simulink model "Copy_of_FaultFeeder"  (R2019a)
settings: Solver=ode1  StartTime=0.0  StopTime=2.5  FixedStep=Ts_Power  RelTol=1e-3
PostLoadFcn:
  | %% Init for wind PnO models - global system parameters
  | OVERRIDE_SSN_MEMORY_LIMIT=1;
  | Ts=50e-6;
  | % Ts=50e-10;
  | Ts_Power=Ts;
  | Ts_Control=2*Ts;
  | freq = 50;
  | Fnom=freq;
  | Vac=400e3;
InitFcn:
  | %% Init for wind PnO models - global system parameters
  | OVERRIDE_SSN_MEMORY_LIMIT=1;
  | Ts=50e-6;
  | % Ts=50e-10;
  | Ts_Power=Ts;
  | Ts_Control=2*Ts;
  | freq = 50;
  | Fnom=freq;
  | Vac=225e3;
values from neighbouring files (symbols this model uses):
  sub_posCap = sub_posCap*2.5    (= 4e-07)    [variable.m]
  sub_posInd = 0.001400563    [variable.m]
  sub_posR = 0.036    [variable.m]
  sub_zeroCap = sub_zeroCap*2.5    (= 1.333325e-07)    [variable.m]
  sub_zeroInd = 0.00420169    [variable.m]
  sub_zeroR = 0.108    [variable.m]
  transfo_L1 = 0.05999374    [variable.m]
  transfo_L2 = 0.05999374    [variable.m]
  transfo_R1 = 0.000866667    [variable.m]
  transfo_R2 = 0.00086667    [variable.m]
undefined symbols (not defined in the file or in its folder): D1, D11, Delta, den, DiscIntNeverNeededParam, dx, find_system, gcbh, num, out_Buses, out_WindFarms, sps_rtmsupport
libraries: powerlib x137, simulink x64, powerlib_meascontrol x64, elements x52, simulink_extras x38, eeSinusoidalMeasurement x35, spsVIMeasurementModel x27, eePowerMeasurement x11
(part 6 of 20)

== system Copy_of_FaultFeeder/SM_WT1/Impedance Element 1/Impedance Relay Scheme ==
  note: Impedance Relay Scheme
  Vabc : Inport
  Iabc : Inport  Port=2
  " 7" : Product  RndMeth=Zero
  "Analog filtering, signal conditioning" : Subsystem
  Combination of Voltages and Currents into 6 pairs (for each type of fault) : Subsystem
  DFT delay : TransportDelay  DelayTime=0.017  BufferSize=30720
  Fault A-B-C Measurement : Subsystem
  Fault A-G Measurement : Subsystem
  Fault B-C Measurement : Subsystem
  Fault B-G Measurement : Subsystem
  Fault C-A Measurement : Subsystem
  Fault C-G Measurement : Subsystem
  Logic Matrix : Subsystem
  Mux{,1,3..6} (6 alike) : Mux
  Mux2 : Mux  Inputs=2
  Product : Product  RndMeth=Zero
  Step1 : Step  Time=0.017  SampleTime=0
  Tripping Logic : Subsystem
  Undervoltage : Subsystem
  tm1 : Terminator
  "TRIP " : Outport  InitialOutput=0  VectorParamsAs1DForOutWhenUnconnected=on
  Logic : Outport  Port=2  InitialOutput=0  VectorParamsAs1DForOutWhenUnconnected=on
  FaultType : Outport  Port=3  InitialOutput=0  VectorParamsAs1DForOutWhenUnconnected=on
  FaultZone : Outport  Port=4  InitialOutput=0  VectorParamsAs1DForOutWhenUnconnected=on
  wires:
  Mux2/1 -> tm1/1
  Tripping Logic/3(Fault Zone) -> FaultZone/1
  Product/1 -> Tripping Logic/5(<V), Fault A-B-C Measurement/2(<V), Fault C-A Measurement/2(<V), Fault B-C Measurement/2(<V), Fault C-G Measurement/2(<V), Fault B-G Measurement/2(<V), Fault A-G Measurement/2(<V)
  Logic Matrix/5(Fault Type) -> FaultType/1
  Tripping Logic/2(Logic Signals) -> Logic/1
  Tripping Logic/1(TRIP) -> "TRIP "/1
  Logic Matrix/4(" Zone4") -> Tripping Logic/4(zone4)
  Logic Matrix/3(" Zone3") -> Tripping Logic/3(zone3)
  Logic Matrix/2(" Zone2") -> Tripping Logic/2(zone2)
  Logic Matrix/1(" Zone1") -> Tripping Logic/1(zone1)
  Mux6/1 -> Logic Matrix/6(A-B-C)
  Mux5/1 -> Logic Matrix/5(C-A)
  Mux4/1 -> Logic Matrix/4(B-C)
  Mux3/1 -> Logic Matrix/3(C-G)
  Mux1/1 -> Logic Matrix/2(B-G)
  Mux/1 -> Logic Matrix/1(A-G)
  Fault A-B-C Measurement/4(Zone4) -> Mux6/4
  Fault A-B-C Measurement/3(Zone3) -> Mux6/3
  Fault A-B-C Measurement/2(Zone2) -> Mux6/2
  Fault A-B-C Measurement/1(Zone1) -> Mux6/1
  Fault C-A Measurement/4(Zone4) -> Mux5/4
  Fault C-A Measurement/3(Zone3) -> Mux5/3
  Fault C-A Measurement/2(Zone2) -> Mux5/2
  Fault C-A Measurement/1(Zone1) -> Mux5/1
  Fault B-C Measurement/4(Zone4) -> Mux4/4
  Fault B-C Measurement/3(Zone3) -> Mux4/3
  Fault B-C Measurement/2(Zone2) -> Mux4/2
  Fault B-C Measurement/1(Zone1) -> Mux4/1
  Fault C-G Measurement/4(Zone4) -> Mux3/4
  Fault C-G Measurement/3(Zone3) -> Mux3/3
  Fault C-G Measurement/2(Zone2) -> Mux3/2
  Fault C-G Measurement/1(Zone1) -> Mux3/1
  Fault B-G Measurement/4(Zone4) -> Mux1/4
  Fault B-G Measurement/3(Zone3) -> Mux1/3
  Fault B-G Measurement/2(Zone2) -> Mux1/2
  Fault B-G Measurement/1(Zone1) -> Mux1/1
  Fault A-G Measurement/4(Zone4) -> Mux/4
  Fault A-G Measurement/3(Zone3) -> Mux/3
  Fault A-G Measurement/2(Zone2) -> Mux/2
  Fault A-G Measurement/1(Zone1) -> Mux/1
  DFT delay/1 -> Product/1
  Combination of Voltages and Currents into 6 pairs (for each type of fault)/6("Volt, Curr A-B,A-B-C-G") -> Fault A-B-C Measurement/1(A-B-C)
  Combination of Voltages and Currents into 6 pairs (for each type of fault)/5("Volt, Curr C-A,C-A-G") -> Fault C-A Measurement/1(C-A)
  Combination of Voltages and Currents into 6 pairs (for each type of fault)/4("Volt, Curr B-C,B-C-G") -> Fault B-C Measurement/1(B-C)
  Combination of Voltages and Currents into 6 pairs (for each type of fault)/3("Volt, Curr C-G") -> Fault C-G Measurement/1(C-G)
  Combination of Voltages and Currents into 6 pairs (for each type of fault)/2("Volt, Curr B-G") -> Fault B-G Measurement/1(B-G)
  "Analog filtering, signal conditioning"/3(If0) -> Combination of Voltages and Currents into 6 pairs (for each type of fault)/3(If0)
  "Analog filtering, signal conditioning"/2(If) -> Combination of Voltages and Currents into 6 pairs (for each type of fault)/2(If)
  "Analog filtering, signal conditioning"/5(if) -> Mux2/2
  "Analog filtering, signal conditioning"/4(vf) -> Mux2/1
  "Analog filtering, signal conditioning"/1(Vf) -> Undervoltage/1("Vabc  "), Combination of Voltages and Currents into 6 pairs (for each type of fault)/1(Vf)
  " 7"/1 -> Product/2, DFT delay/1
  Step1/1 -> " 7"/2
  Undervoltage/1(<V) -> " 7"/1
  Combination of Voltages and Currents into 6 pairs (for each type of fault)/1("Volt, Curr A-G") -> Fault A-G Measurement/1(A-G)
  Iabc/1 -> "Analog filtering, signal conditioning"/2(Iin)
  Vabc/1 -> "Analog filtering, signal conditioning"/1(Vin)

== system Copy_of_FaultFeeder/SM_WT1/Impedance Element 2/Impedance Relay Scheme ==
  note: Impedance Relay Scheme
  Vabc : Inport
  Iabc : Inport  Port=2
  " 7" : Product  RndMeth=Zero
  "Analog filtering, signal conditioning" : Subsystem
  Combination of Voltages and Currents into 6 pairs (for each type of fault) : Subsystem
  DFT delay : TransportDelay  DelayTime=0.017  BufferSize=30720
  Fault A-B-C Measurement : Subsystem
  Fault A-G Measurement : Subsystem
  Fault B-C Measurement : Subsystem
  Fault B-G Measurement : Subsystem
  Fault C-A Measurement : Subsystem
  Fault C-G Measurement : Subsystem
  Logic Matrix : Subsystem
  Mux{,1,3..6} (6 alike) : Mux
  Mux2 : Mux  Inputs=2
  Product : Product  RndMeth=Zero
  Step1 : Step  Time=0.017  SampleTime=0
  Tripping Logic : Subsystem
  Undervoltage : Subsystem
  tm1 : Terminator
  "TRIP " : Outport  InitialOutput=0  VectorParamsAs1DForOutWhenUnconnected=on
  Logic : Outport  Port=2  InitialOutput=0  VectorParamsAs1DForOutWhenUnconnected=on
  FaultType : Outport  Port=3  InitialOutput=0  VectorParamsAs1DForOutWhenUnconnected=on
  FaultZone : Outport  Port=4  InitialOutput=0  VectorParamsAs1DForOutWhenUnconnected=on
  wires:
  Mux2/1 -> tm1/1
  Tripping Logic/3(Fault Zone) -> FaultZone/1
  Product/1 -> Tripping Logic/5(<V), Fault A-B-C Measurement/2(<V), Fault C-A Measurement/2(<V), Fault B-C Measurement/2(<V), Fault C-G Measurement/2(<V), Fault B-G Measurement/2(<V), Fault A-G Measurement/2(<V)
  Logic Matrix/5(Fault Type) -> FaultType/1
  Tripping Logic/2(Logic Signals) -> Logic/1
  Tripping Logic/1(TRIP) -> "TRIP "/1
  Logic Matrix/4(" Zone4") -> Tripping Logic/4(zone4)
  Logic Matrix/3(" Zone3") -> Tripping Logic/3(zone3)
  Logic Matrix/2(" Zone2") -> Tripping Logic/2(zone2)
  Logic Matrix/1(" Zone1") -> Tripping Logic/1(zone1)
  Mux6/1 -> Logic Matrix/6(A-B-C)
  Mux5/1 -> Logic Matrix/5(C-A)
  Mux4/1 -> Logic Matrix/4(B-C)
  Mux3/1 -> Logic Matrix/3(C-G)
  Mux1/1 -> Logic Matrix/2(B-G)
  Mux/1 -> Logic Matrix/1(A-G)
  Fault A-B-C Measurement/4(Zone4) -> Mux6/4
  Fault A-B-C Measurement/3(Zone3) -> Mux6/3
  Fault A-B-C Measurement/2(Zone2) -> Mux6/2
  Fault A-B-C Measurement/1(Zone1) -> Mux6/1
  Fault C-A Measurement/4(Zone4) -> Mux5/4
  Fault C-A Measurement/3(Zone3) -> Mux5/3
  Fault C-A Measurement/2(Zone2) -> Mux5/2
  Fault C-A Measurement/1(Zone1) -> Mux5/1
  Fault B-C Measurement/4(Zone4) -> Mux4/4
  Fault B-C Measurement/3(Zone3) -> Mux4/3
  Fault B-C Measurement/2(Zone2) -> Mux4/2
  Fault B-C Measurement/1(Zone1) -> Mux4/1
  Fault C-G Measurement/4(Zone4) -> Mux3/4
  Fault C-G Measurement/3(Zone3) -> Mux3/3
  Fault C-G Measurement/2(Zone2) -> Mux3/2
  Fault C-G Measurement/1(Zone1) -> Mux3/1
  Fault B-G Measurement/4(Zone4) -> Mux1/4
  Fault B-G Measurement/3(Zone3) -> Mux1/3
  Fault B-G Measurement/2(Zone2) -> Mux1/2
  Fault B-G Measurement/1(Zone1) -> Mux1/1
  Fault A-G Measurement/4(Zone4) -> Mux/4
  Fault A-G Measurement/3(Zone3) -> Mux/3
  Fault A-G Measurement/2(Zone2) -> Mux/2
  Fault A-G Measurement/1(Zone1) -> Mux/1
  DFT delay/1 -> Product/1
  Combination of Voltages and Currents into 6 pairs (for each type of fault)/6("Volt, Curr A-B,A-B-C-G") -> Fault A-B-C Measurement/1(A-B-C)
  Combination of Voltages and Currents into 6 pairs (for each type of fault)/5("Volt, Curr C-A,C-A-G") -> Fault C-A Measurement/1(C-A)
  Combination of Voltages and Currents into 6 pairs (for each type of fault)/4("Volt, Curr B-C,B-C-G") -> Fault B-C Measurement/1(B-C)
  Combination of Voltages and Currents into 6 pairs (for each type of fault)/3("Volt, Curr C-G") -> Fault C-G Measurement/1(C-G)
  Combination of Voltages and Currents into 6 pairs (for each type of fault)/2("Volt, Curr B-G") -> Fault B-G Measurement/1(B-G)
  "Analog filtering, signal conditioning"/3(If0) -> Combination of Voltages and Currents into 6 pairs (for each type of fault)/3(If0)
  "Analog filtering, signal conditioning"/2(If) -> Combination of Voltages and Currents into 6 pairs (for each type of fault)/2(If)
  "Analog filtering, signal conditioning"/5(if) -> Mux2/2
  "Analog filtering, signal conditioning"/4(vf) -> Mux2/1
  "Analog filtering, signal conditioning"/1(Vf) -> Undervoltage/1("Vabc  "), Combination of Voltages and Currents into 6 pairs (for each type of fault)/1(Vf)
  " 7"/1 -> Product/2, DFT delay/1
  Step1/1 -> " 7"/2
  Undervoltage/1(<V) -> " 7"/1
  Combination of Voltages and Currents into 6 pairs (for each type of fault)/1("Volt, Curr A-G") -> Fault A-G Measurement/1(A-G)
  Iabc/1 -> "Analog filtering, signal conditioning"/2(Iin)
  Vabc/1 -> "Analog filtering, signal conditioning"/1(Vin)

== system Copy_of_FaultFeeder/SM_WT1/Overcurrent Element 1/Overcurrent Relay Scheme ==
  note: Overcurrent Relay Scheme
  Iabc : Inport
  "Analog filtering, signal conditioning" : Subsystem
  Data Type Conversion : DataTypeConversion  OutDataTypeStr=double
  Demux : Demux  Outputs=3
  Logic Matrix : Subsystem
  Phase A : Subsystem
  Phase B : Subsystem
  Phase C : Subsystem
  Residual : Subsystem
  Scope : Scope
  Tripping Logic : Subsystem
  tm1 : Terminator
  "TRIP " : Outport  InitialOutput=0  VectorParamsAs1DForOutWhenUnconnected=on
  Logic : Outport  Port=2  InitialOutput=0  VectorParamsAs1DForOutWhenUnconnected=on
  FaultType : Outport  Port=3  InitialOutput=0  VectorParamsAs1DForOutWhenUnconnected=on
  wires:
  Iabc/1 -> "Analog filtering, signal conditioning"/1(Iin)
  Tripping Logic/1(TRIP) -> "TRIP "/1
  Tripping Logic/2(Logic Signals) -> Logic/1
  "Analog filtering, signal conditioning"/1(If) -> Scope/1, Demux/1
  Demux/1 -> Phase A/1(IA)
  "Analog filtering, signal conditioning"/2(If0) -> Residual/1(IR)
  Demux/2 -> Phase B/1(IB)
  Demux/3 -> Phase C/1(IC)
  Phase A/1(Pickup) -> Logic Matrix/1(A)
  Phase B/1(Pickup) -> Logic Matrix/2(B)
  Phase C/1(Pickup) -> Logic Matrix/3(C)
  Residual/1(Pickup) -> Logic Matrix/4(R), Data Type Conversion/1
  Logic Matrix/1(" Op") -> Tripping Logic/1(Op)
  Logic Matrix/2(Fault Type) -> FaultType/1
  "Analog filtering, signal conditioning"/3(if) -> tm1/1
  Data Type Conversion/1 -> Tripping Logic/2(IR)

== system Copy_of_FaultFeeder/SM_WT1/Overcurrent Element 2/Overcurrent Relay Scheme ==
  note: Overcurrent Relay Scheme
  Iabc : Inport
  "Analog filtering, signal conditioning" : Subsystem
  Data Type Conversion : DataTypeConversion  OutDataTypeStr=double
  Demux : Demux  Outputs=3
  Logic Matrix : Subsystem
  Phase A : Subsystem
  Phase B : Subsystem
  Phase C : Subsystem
  Residual : Subsystem
  Tripping Logic : Subsystem
  tm1 : Terminator
  "TRIP " : Outport  InitialOutput=0  VectorParamsAs1DForOutWhenUnconnected=on
  Logic : Outport  Port=2  InitialOutput=0  VectorParamsAs1DForOutWhenUnconnected=on
  FaultType : Outport  Port=3  InitialOutput=0  VectorParamsAs1DForOutWhenUnconnected=on
  wires:
  Iabc/1 -> "Analog filtering, signal conditioning"/1(Iin)
  Tripping Logic/1(TRIP) -> "TRIP "/1
  Tripping Logic/2(Logic Signals) -> Logic/1
  "Analog filtering, signal conditioning"/1(If) -> Demux/1
  Demux/1 -> Phase A/1(IA)
  "Analog filtering, signal conditioning"/2(If0) -> Residual/1(IR)
  Demux/2 -> Phase B/1(IB)
  Demux/3 -> Phase C/1(IC)
  Phase A/1(Pickup) -> Logic Matrix/1(A)
  Phase B/1(Pickup) -> Logic Matrix/2(B)
  Phase C/1(Pickup) -> Logic Matrix/3(C)
  Residual/1(Pickup) -> Logic Matrix/4(R), Data Type Conversion/1
  Logic Matrix/1(" Op") -> Tripping Logic/1(Op)
  Logic Matrix/2(Fault Type) -> FaultType/1
  "Analog filtering, signal conditioning"/3(if) -> tm1/1
  Data Type Conversion/1 -> Tripping Logic/2(IR)

== system Copy_of_FaultFeeder/SM_WT1/Overcurrent Inverse time/Overcurrent Relay Scheme ==
  note: Overcurrent Relay Scheme
  Iabc : Inport
  "Analog filtering, signal conditioning" : Subsystem
  Demux : Demux  Outputs=3
  Logic Matrix : Subsystem
  Phase A : Subsystem
  Phase B : Subsystem
  Phase C : Subsystem
  Tripping Logic : Subsystem
  tm1 : Terminator
  tm2 : Terminator
  "TRIP " : Outport  InitialOutput=0  VectorParamsAs1DForOutWhenUnconnected=on
  FaultType : Outport  Port=2  InitialOutput=0  VectorParamsAs1DForOutWhenUnconnected=on
  wires:
  Tripping Logic/1(TRIP) -> "TRIP "/1
  "Analog filtering, signal conditioning"/1(If) -> Demux/1
  Demux/1 -> Phase A/1(IA)
  Demux/2 -> Phase B/1(IB)
  Demux/3 -> Phase C/1(IC)
  Phase A/1(Pickup) -> Logic Matrix/1(A)
  Phase B/1(Pickup) -> Logic Matrix/2(B)
  Phase C/1(Pickup) -> Logic Matrix/3(C)
  Logic Matrix/1(" Op") -> Tripping Logic/1(Op)
  Logic Matrix/2(Fault Type) -> FaultType/1
  "Analog filtering, signal conditioning"/3(if) -> tm1/1
  "Analog filtering, signal conditioning"/2(If0) -> tm2/1
  Iabc/1 -> "Analog filtering, signal conditioning"/1(Iin)

== system Copy_of_FaultFeeder/SM_WT1/Subsystem1/Subsystem ==
  V : Inport
  I : Inport  Port=2
  Bus Creator : BusCreator  Inputs=2
  Gain : Gain  Gain=1/1e6
  Gain1 : Gain  Gain=1/1e6
  Gain2 : Gain  Gain=1/1e3
  Gain3 : Gain  Gain=1/1e3
  Power Measurement (Three-Phase) : eePowerMeasurement/Power Measurement (Three-Phase)  LabelModeActiveChoice=Discrete  F=freq  K=1  Seq=Positive  Ts=Ts
      settings: SourceProductBaseCode=PS
  "Sinusoidal Measurement (PLL, Three-Phase)1" : eeSinusoidalMeasurement/Sinusoidal Measurement (PLL, Three-Phase)  Kp_LF=200  Ki_LF=2000  F0=freq  Theta0=0  Ts=-1
      settings: SourceProductBaseCode=PS
  "Sinusoidal Measurement (PLL, Three-Phase)6" : eeSinusoidalMeasurement/Sinusoidal Measurement (PLL, Three-Phase)  Kp_LF=200  Ki_LF=2000  F0=freq  Theta0=0  Ts=-1
      settings: SourceProductBaseCode=PS
  Terminator{,1..3} (4 alike) : Terminator
  Vabc : Outport  VectorParamsAs1DForOutWhenUnconnected=on
  Iabc : Outport  Port=2  VectorParamsAs1DForOutWhenUnconnected=on
  V mag : Outport  Port=3  VectorParamsAs1DForOutWhenUnconnected=on
  I mag : Outport  Port=4  VectorParamsAs1DForOutWhenUnconnected=on
  PQ : Outport  Port=5  VectorParamsAs1DForOutWhenUnconnected=on
  wires:
  Gain3/1 -> V mag/1  "V (kV)"
  I/1 -> Iabc/1, "Sinusoidal Measurement (PLL, Three-Phase)1"/1, Power Measurement (Three-Phase)/2  "I (A)"
  Power Measurement (Three-Phase)/1 -> Gain/1  "P (W)"
  Gain/1 -> Bus Creator/1  "P (MW)"
  Power Measurement (Three-Phase)/2 -> Gain1/1  "Q (VAr)"
  Bus Creator/1 -> PQ/1  "PQ"
  Gain1/1 -> Bus Creator/2  "Q (MVAr)"
  Gain2/1 -> Vabc/1  "V (kV)"
  V/1 -> Power Measurement (Three-Phase)/1, Gain2/1, "Sinusoidal Measurement (PLL, Three-Phase)6"/1  "V (V)"
  "Sinusoidal Measurement (PLL, Three-Phase)6"/2 -> Terminator/1
  "Sinusoidal Measurement (PLL, Three-Phase)6"/1 -> Terminator1/1
  "Sinusoidal Measurement (PLL, Three-Phase)6"/3 -> Gain3/1
  "Sinusoidal Measurement (PLL, Three-Phase)1"/3 -> I mag/1
  "Sinusoidal Measurement (PLL, Three-Phase)1"/1 -> Terminator3/1
  "Sinusoidal Measurement (PLL, Three-Phase)1"/2 -> Terminator2/1

== system Copy_of_FaultFeeder/SM_WT1/Subsystem2/Subsystem ==
  V : Inport
  I : Inport  Port=2
  Bus Creator : BusCreator  Inputs=2
  Gain : Gain  Gain=1/1e6
  Gain1 : Gain  Gain=1/1e6
  Gain2 : Gain  Gain=1/1e3
  Gain3 : Gain  Gain=1/1e3
  Power Measurement (Three-Phase) : eePowerMeasurement/Power Measurement (Three-Phase)  LabelModeActiveChoice=Discrete  F=freq  K=1  Seq=Positive  Ts=Ts
      settings: SourceProductBaseCode=PS
  "Sinusoidal Measurement (PLL, Three-Phase)1" : eeSinusoidalMeasurement/Sinusoidal Measurement (PLL, Three-Phase)  Kp_LF=200  Ki_LF=2000  F0=freq  Theta0=0  Ts=-1
      settings: SourceProductBaseCode=PS
  "Sinusoidal Measurement (PLL, Three-Phase)6" : eeSinusoidalMeasurement/Sinusoidal Measurement (PLL, Three-Phase)  Kp_LF=200  Ki_LF=2000  F0=freq  Theta0=0  Ts=-1
      settings: SourceProductBaseCode=PS
  Terminator{,1..3} (4 alike) : Terminator
  Vabc : Outport  VectorParamsAs1DForOutWhenUnconnected=on
  Iabc : Outport  Port=2  VectorParamsAs1DForOutWhenUnconnected=on
  V mag : Outport  Port=3  VectorParamsAs1DForOutWhenUnconnected=on
  I mag : Outport  Port=4  VectorParamsAs1DForOutWhenUnconnected=on
  PQ : Outport  Port=5  VectorParamsAs1DForOutWhenUnconnected=on
  wires:
  "Sinusoidal Measurement (PLL, Three-Phase)1"/2 -> Terminator2/1
  "Sinusoidal Measurement (PLL, Three-Phase)1"/1 -> Terminator3/1
  "Sinusoidal Measurement (PLL, Three-Phase)1"/3 -> I mag/1
  "Sinusoidal Measurement (PLL, Three-Phase)6"/3 -> Gain3/1
  "Sinusoidal Measurement (PLL, Three-Phase)6"/1 -> Terminator1/1
  "Sinusoidal Measurement (PLL, Three-Phase)6"/2 -> Terminator/1
  V/1 -> "Sinusoidal Measurement (PLL, Three-Phase)6"/1, Gain2/1, Power Measurement (Three-Phase)/1  "V (V)"
  Gain2/1 -> Vabc/1  "V (kV)"
  Gain1/1 -> Bus Creator/2  "Q (MVAr)"
  Bus Creator/1 -> PQ/1  "PQ"
  Power Measurement (Three-Phase)/2 -> Gain1/1  "Q (VAr)"
  Gain/1 -> Bus Creator/1  "P (MW)"
  Power Measurement (Three-Phase)/1 -> Gain/1  "P (W)"
  I/1 -> Power Measurement (Three-Phase)/2, "Sinusoidal Measurement (PLL, Three-Phase)1"/1, Iabc/1  "I (A)"
  Gain3/1 -> V mag/1  "V (kV)"

== system Copy_of_FaultFeeder/SM_WT1/Subsystem3/Subsystem ==
  V : Inport
  I : Inport  Port=2
  Bus Creator : BusCreator  Inputs=2
  Gain : Gain  Gain=1/1e6
  Gain1 : Gain  Gain=1/1e6
  Gain2 : Gain  Gain=1/1e3
  Gain3 : Gain  Gain=1/1e3
  Power Measurement (Three-Phase) : eePowerMeasurement/Power Measurement (Three-Phase)  LabelModeActiveChoice=Discrete  F=freq  K=1  Seq=Positive  Ts=Ts
      settings: SourceProductBaseCode=PS
  "Sinusoidal Measurement (PLL, Three-Phase)1" : eeSinusoidalMeasurement/Sinusoidal Measurement (PLL, Three-Phase)  Kp_LF=200  Ki_LF=2000  F0=freq  Theta0=0  Ts=-1
      settings: SourceProductBaseCode=PS
  "Sinusoidal Measurement (PLL, Three-Phase)6" : eeSinusoidalMeasurement/Sinusoidal Measurement (PLL, Three-Phase)  Kp_LF=200  Ki_LF=2000  F0=freq  Theta0=0  Ts=-1
      settings: SourceProductBaseCode=PS
  Terminator{,1..3} (4 alike) : Terminator
  Vabc : Outport  VectorParamsAs1DForOutWhenUnconnected=on
  Iabc : Outport  Port=2  VectorParamsAs1DForOutWhenUnconnected=on
  V mag : Outport  Port=3  VectorParamsAs1DForOutWhenUnconnected=on
  I mag : Outport  Port=4  VectorParamsAs1DForOutWhenUnconnected=on
  PQ : Outport  Port=5  VectorParamsAs1DForOutWhenUnconnected=on
  wires:
  "Sinusoidal Measurement (PLL, Three-Phase)1"/2 -> Terminator2/1
  "Sinusoidal Measurement (PLL, Three-Phase)1"/1 -> Terminator3/1
  "Sinusoidal Measurement (PLL, Three-Phase)1"/3 -> I mag/1
  "Sinusoidal Measurement (PLL, Three-Phase)6"/3 -> Gain3/1
  "Sinusoidal Measurement (PLL, Three-Phase)6"/1 -> Terminator1/1
  "Sinusoidal Measurement (PLL, Three-Phase)6"/2 -> Terminator/1
  V/1 -> "Sinusoidal Measurement (PLL, Three-Phase)6"/1, Gain2/1, Power Measurement (Three-Phase)/1  "V (V)"
  Gain2/1 -> Vabc/1  "V (kV)"
  Gain1/1 -> Bus Creator/2  "Q (MVAr)"
  Bus Creator/1 -> PQ/1  "PQ"
  Power Measurement (Three-Phase)/2 -> Gain1/1  "Q (VAr)"
  Gain/1 -> Bus Creator/1  "P (MW)"
  Power Measurement (Three-Phase)/1 -> Gain/1  "P (W)"
  I/1 -> Power Measurement (Three-Phase)/2, "Sinusoidal Measurement (PLL, Three-Phase)1"/1, Iabc/1  "I (A)"
  Gain3/1 -> V mag/1  "V (kV)"

== system Copy_of_FaultFeeder/SM_WT1/Subsystem4/Subsystem ==
  V : Inport
  I : Inport  Port=2
  Bus Creator : BusCreator  Inputs=2
  Gain : Gain  Gain=1/1e6
  Gain1 : Gain  Gain=1/1e6
  Gain2 : Gain  Gain=1/1e3
  Gain3 : Gain  Gain=1/1e3
  Power Measurement (Three-Phase) : eePowerMeasurement/Power Measurement (Three-Phase)  LabelModeActiveChoice=Discrete  F=freq  K=1  Seq=Positive  Ts=Ts
      settings: SourceProductBaseCode=PS
  "Sinusoidal Measurement (PLL, Three-Phase)1" : eeSinusoidalMeasurement/Sinusoidal Measurement (PLL, Three-Phase)  Kp_LF=200  Ki_LF=2000  F0=freq  Theta0=0  Ts=-1
      settings: SourceProductBaseCode=PS
  "Sinusoidal Measurement (PLL, Three-Phase)6" : eeSinusoidalMeasurement/Sinusoidal Measurement (PLL, Three-Phase)  Kp_LF=200  Ki_LF=2000  F0=freq  Theta0=0  Ts=-1
      settings: SourceProductBaseCode=PS
  Terminator{,1..3} (4 alike) : Terminator
  Vabc : Outport  VectorParamsAs1DForOutWhenUnconnected=on
  Iabc : Outport  Port=2  VectorParamsAs1DForOutWhenUnconnected=on
  V mag : Outport  Port=3  VectorParamsAs1DForOutWhenUnconnected=on
  I mag : Outport  Port=4  VectorParamsAs1DForOutWhenUnconnected=on
  PQ : Outport  Port=5  VectorParamsAs1DForOutWhenUnconnected=on
  wires:
  Gain3/1 -> V mag/1  "V (kV)"
  I/1 -> Iabc/1, "Sinusoidal Measurement (PLL, Three-Phase)1"/1, Power Measurement (Three-Phase)/2  "I (A)"
  Power Measurement (Three-Phase)/1 -> Gain/1  "P (W)"
  Gain/1 -> Bus Creator/1  "P (MW)"
  Power Measurement (Three-Phase)/2 -> Gain1/1  "Q (VAr)"
  Bus Creator/1 -> PQ/1  "PQ"
  Gain1/1 -> Bus Creator/2  "Q (MVAr)"
  Gain2/1 -> Vabc/1  "V (kV)"
  V/1 -> Power Measurement (Three-Phase)/1, Gain2/1, "Sinusoidal Measurement (PLL, Three-Phase)6"/1  "V (V)"
  "Sinusoidal Measurement (PLL, Three-Phase)6"/2 -> Terminator/1
  "Sinusoidal Measurement (PLL, Three-Phase)6"/1 -> Terminator1/1
  "Sinusoidal Measurement (PLL, Three-Phase)6"/3 -> Gain3/1
  "Sinusoidal Measurement (PLL, Three-Phase)1"/3 -> I mag/1
  "Sinusoidal Measurement (PLL, Three-Phase)1"/1 -> Terminator3/1
  "Sinusoidal Measurement (PLL, Three-Phase)1"/2 -> Terminator2/1

== system Copy_of_FaultFeeder/SM_WT1/Subsystem5/Subsystem ==
  V : Inport
  I : Inport  Port=2
  Bus Creator : BusCreator  Inputs=2
  Gain : Gain  Gain=1/1e6
  Gain1 : Gain  Gain=1/1e6
  Gain2 : Gain  Gain=1/1e3
  Gain3 : Gain  Gain=1/1e3
  Power Measurement (Three-Phase) : eePowerMeasurement/Power Measurement (Three-Phase)  LabelModeActiveChoice=Discrete  F=freq  K=1  Seq=Positive  Ts=Ts
      settings: SourceProductBaseCode=PS
  "Sinusoidal Measurement (PLL, Three-Phase)1" : eeSinusoidalMeasurement/Sinusoidal Measurement (PLL, Three-Phase)  Kp_LF=200  Ki_LF=2000  F0=freq  Theta0=0  Ts=-1
      settings: SourceProductBaseCode=PS
  "Sinusoidal Measurement (PLL, Three-Phase)6" : eeSinusoidalMeasurement/Sinusoidal Measurement (PLL, Three-Phase)  Kp_LF=200  Ki_LF=2000  F0=freq  Theta0=0  Ts=-1
      settings: SourceProductBaseCode=PS
  Terminator{,1..3} (4 alike) : Terminator
  Vabc : Outport  VectorParamsAs1DForOutWhenUnconnected=on
  Iabc : Outport  Port=2  VectorParamsAs1DForOutWhenUnconnected=on
  V mag : Outport  Port=3  VectorParamsAs1DForOutWhenUnconnected=on
  I mag : Outport  Port=4  VectorParamsAs1DForOutWhenUnconnected=on
  PQ : Outport  Port=5  VectorParamsAs1DForOutWhenUnconnected=on
  wires:
  "Sinusoidal Measurement (PLL, Three-Phase)1"/2 -> Terminator2/1
  "Sinusoidal Measurement (PLL, Three-Phase)1"/1 -> Terminator3/1
  "Sinusoidal Measurement (PLL, Three-Phase)1"/3 -> I mag/1
  "Sinusoidal Measurement (PLL, Three-Phase)6"/3 -> Gain3/1
  "Sinusoidal Measurement (PLL, Three-Phase)6"/1 -> Terminator1/1
  "Sinusoidal Measurement (PLL, Three-Phase)6"/2 -> Terminator/1
  V/1 -> "Sinusoidal Measurement (PLL, Three-Phase)6"/1, Gain2/1, Power Measurement (Three-Phase)/1  "V (V)"
  Gain2/1 -> Vabc/1  "V (kV)"
  Gain1/1 -> Bus Creator/2  "Q (MVAr)"
  Bus Creator/1 -> PQ/1  "PQ"
  Power Measurement (Three-Phase)/2 -> Gain1/1  "Q (VAr)"
  Gain/1 -> Bus Creator/1  "P (MW)"
  Power Measurement (Three-Phase)/1 -> Gain/1  "P (W)"
  I/1 -> Power Measurement (Three-Phase)/2, "Sinusoidal Measurement (PLL, Three-Phase)1"/1, Iabc/1  "I (A)"
  Gain3/1 -> V mag/1  "V (kV)"

== system Copy_of_FaultFeeder/SM_WT1/Subsystem6/Subsystem ==
  V : Inport
  I : Inport  Port=2
  Bus Creator : BusCreator  Inputs=2
  Gain : Gain  Gain=1/1e6
  Gain1 : Gain  Gain=1/1e6
  Gain2 : Gain  Gain=1/1e3
  Gain3 : Gain  Gain=1/1e3
  Power Measurement (Three-Phase) : eePowerMeasurement/Power Measurement (Three-Phase)  LabelModeActiveChoice=Discrete  F=freq  K=1  Seq=Positive  Ts=Ts
      settings: SourceProductBaseCode=PS
  "Sinusoidal Measurement (PLL, Three-Phase)1" : eeSinusoidalMeasurement/Sinusoidal Measurement (PLL, Three-Phase)  Kp_LF=200  Ki_LF=2000  F0=freq  Theta0=0  Ts=-1
      settings: SourceProductBaseCode=PS
  "Sinusoidal Measurement (PLL, Three-Phase)6" : eeSinusoidalMeasurement/Sinusoidal Measurement (PLL, Three-Phase)  Kp_LF=200  Ki_LF=2000  F0=freq  Theta0=0  Ts=-1
      settings: SourceProductBaseCode=PS
  Terminator{,1..3} (4 alike) : Terminator
  Vabc : Outport  VectorParamsAs1DForOutWhenUnconnected=on
  Iabc : Outport  Port=2  VectorParamsAs1DForOutWhenUnconnected=on
  V mag : Outport  Port=3  VectorParamsAs1DForOutWhenUnconnected=on
  I mag : Outport  Port=4  VectorParamsAs1DForOutWhenUnconnected=on
  PQ : Outport  Port=5  VectorParamsAs1DForOutWhenUnconnected=on
  wires:
  "Sinusoidal Measurement (PLL, Three-Phase)1"/2 -> Terminator2/1
  "Sinusoidal Measurement (PLL, Three-Phase)1"/1 -> Terminator3/1
  "Sinusoidal Measurement (PLL, Three-Phase)1"/3 -> I mag/1
  "Sinusoidal Measurement (PLL, Three-Phase)6"/3 -> Gain3/1
  "Sinusoidal Measurement (PLL, Three-Phase)6"/1 -> Terminator1/1
  "Sinusoidal Measurement (PLL, Three-Phase)6"/2 -> Terminator/1
  V/1 -> "Sinusoidal Measurement (PLL, Three-Phase)6"/1, Gain2/1, Power Measurement (Three-Phase)/1  "V (V)"
  Gain2/1 -> Vabc/1  "V (kV)"
  Gain1/1 -> Bus Creator/2  "Q (MVAr)"
  Bus Creator/1 -> PQ/1  "PQ"
  Power Measurement (Three-Phase)/2 -> Gain1/1  "Q (VAr)"
  Gain/1 -> Bus Creator/1  "P (MW)"
  Power Measurement (Three-Phase)/1 -> Gain/1  "P (W)"
  I/1 -> Power Measurement (Three-Phase)/2, "Sinusoidal Measurement (PLL, Three-Phase)1"/1, Iabc/1  "I (A)"
  Gain3/1 -> V mag/1  "V (kV)"

== system Copy_of_FaultFeeder/SM_WT1/Subsystem9/Subsystem ==
  V : Inport
  I : Inport  Port=2
  Bus Creator : BusCreator  Inputs=2
  Gain : Gain  Gain=1/1e6
  Gain1 : Gain  Gain=1/1e6
  Gain2 : Gain  Gain=1/1e3
  Gain3 : Gain  Gain=1/1e3
  Power Measurement (Three-Phase) : eePowerMeasurement/Power Measurement (Three-Phase)  LabelModeActiveChoice=Discrete  F=freq  K=1  Seq=Positive  Ts=Ts
      settings: SourceProductBaseCode=PS
  "Sinusoidal Measurement (PLL, Three-Phase)1" : eeSinusoidalMeasurement/Sinusoidal Measurement (PLL, Three-Phase)  Kp_LF=200  Ki_LF=2000  F0=freq  Theta0=0  Ts=-1
      settings: SourceProductBaseCode=PS
  "Sinusoidal Measurement (PLL, Three-Phase)6" : eeSinusoidalMeasurement/Sinusoidal Measurement (PLL, Three-Phase)  Kp_LF=200  Ki_LF=2000  F0=freq  Theta0=0  Ts=-1
      settings: SourceProductBaseCode=PS
  Terminator{,1..3} (4 alike) : Terminator
  Vabc : Outport  VectorParamsAs1DForOutWhenUnconnected=on
  Iabc : Outport  Port=2  VectorParamsAs1DForOutWhenUnconnected=on
  V mag : Outport  Port=3  VectorParamsAs1DForOutWhenUnconnected=on
  I mag : Outport  Port=4  VectorParamsAs1DForOutWhenUnconnected=on
  PQ : Outport  Port=5  VectorParamsAs1DForOutWhenUnconnected=on
  wires:
  "Sinusoidal Measurement (PLL, Three-Phase)1"/2 -> Terminator2/1
  "Sinusoidal Measurement (PLL, Three-Phase)1"/1 -> Terminator3/1
  "Sinusoidal Measurement (PLL, Three-Phase)1"/3 -> I mag/1
  "Sinusoidal Measurement (PLL, Three-Phase)6"/3 -> Gain3/1
  "Sinusoidal Measurement (PLL, Three-Phase)6"/1 -> Terminator1/1
  "Sinusoidal Measurement (PLL, Three-Phase)6"/2 -> Terminator/1
  V/1 -> "Sinusoidal Measurement (PLL, Three-Phase)6"/1, Gain2/1, Power Measurement (Three-Phase)/1  "V (V)"
  Gain2/1 -> Vabc/1  "V (kV)"
  Gain1/1 -> Bus Creator/2  "Q (MVAr)"
  Bus Creator/1 -> PQ/1  "PQ"
  Power Measurement (Three-Phase)/2 -> Gain1/1  "Q (VAr)"
  Gain/1 -> Bus Creator/1  "P (MW)"
  Power Measurement (Three-Phase)/1 -> Gain/1  "P (W)"
  I/1 -> Power Measurement (Three-Phase)/2, "Sinusoidal Measurement (PLL, Three-Phase)1"/1, Iabc/1  "I (A)"
  Gain3/1 -> V mag/1  "V (kV)"

== system Copy_of_FaultFeeder/SM_WT1/Transformer differential element 1/Differential Relay ==
  IDa1 : Inport
  IDa2 : Inport  Port=2
  IDa5 : Inport  Port=3
  IDb1 : Inport  Port=4
  IDb2 : Inport  Port=5
  IDb5 : Inport  Port=6
  IDc1 : Inport  Port=7
  IDc2 : Inport  Port=8
  IDc5 : Inport  Port=9
  IRa1 : Inport  Port=10
  IRb1 : Inport  Port=11
  IRc1 : Inport  Port=12
  Logical Operator : Logic  Operator=OR  Inputs=3
  logic block : Subsystem
  logic block1 : Subsystem
  logic block2 : Subsystem
  Trip1 : Outport  VectorParamsAs1DForOutWhenUnconnected=on
  wires:
  logic block/1(Trip A) -> Logical Operator/1
  logic block2/1(Trip C) -> Logical Operator/3
  Logical Operator/1 -> Trip1/1
  IRc1/1 -> logic block2/2(IRc1)
  IRb1/1 -> logic block1/2(IRb1)
  IDc5/1 -> logic block2/4(IDc5)
  IDc2/1 -> logic block2/3(IDc2)
  IDb2/1 -> logic block1/3(IDb2)
  IDb1/1 -> logic block1/1(IDb1)
  IDa5/1 -> logic block/4(IDa5)
  IDa2/1 -> logic block/3(IDa2)
  IDa1/1 -> logic block/1(IDa1)
  IRa1/1 -> logic block/2(IRa1)
  IDc1/1 -> logic block2/1(IDc1)
  IDb5/1 -> logic block1/4(IDb5)
  logic block1/1(Trip B) -> Logical Operator/2

== system Copy_of_FaultFeeder/SM_WT1/Transformer differential element 1/Signal Processing1 ==
  IHA : Inport
  IHB : Inport  Port=2
  IHC : Inport  Port=3
  IXA : Inport  Port=4
  IXB : Inport  Port=5
  IXC : Inport  Port=6
  Differential and restraining currents : Subsystem
  Phasor-magnitude (IR) : Subsystem
  phasor-magnitude (IDa) : Subsystem
  phasor-magnitude (iDb) : Subsystem
  phasor-magnitude (iDc) : Subsystem
  iDa1 : Outport  VectorParamsAs1DForOutWhenUnconnected=on
  iDa2 : Outport  Port=2  VectorParamsAs1DForOutWhenUnconnected=on
  iDa5 : Outport  Port=3  VectorParamsAs1DForOutWhenUnconnected=on
  iDb1 : Outport  Port=4  VectorParamsAs1DForOutWhenUnconnected=on
  iDb2 : Outport  Port=5  VectorParamsAs1DForOutWhenUnconnected=on
  iDb5 : Outport  Port=6  VectorParamsAs1DForOutWhenUnconnected=on
  iDc1 : Outport  Port=7  VectorParamsAs1DForOutWhenUnconnected=on
  iDc2 : Outport  Port=8  VectorParamsAs1DForOutWhenUnconnected=on
  iDc5 : Outport  Port=9  VectorParamsAs1DForOutWhenUnconnected=on
  iRa1 : Outport  Port=10  VectorParamsAs1DForOutWhenUnconnected=on
  iRb1 : Outport  Port=11  VectorParamsAs1DForOutWhenUnconnected=on
  iRc1 : Outport  Port=12  VectorParamsAs1DForOutWhenUnconnected=on
  wires:
  IHA/1 -> Differential and restraining currents/1(IHA)
  IHB/1 -> Differential and restraining currents/2(IHB)
  IHC/1 -> Differential and restraining currents/3(IHC)
  IXA/1 -> Differential and restraining currents/4(IXA)
  IXB/1 -> Differential and restraining currents/5(IXB)
  IXC/1 -> Differential and restraining currents/6(IXC)
  Differential and restraining currents/1(iDa1) -> phasor-magnitude (IDa)/1(In1)
  Differential and restraining currents/2(iDa2) -> phasor-magnitude (IDa)/2(In2)
  Differential and restraining currents/3(iDa5) -> phasor-magnitude (IDa)/3(In3)
  phasor-magnitude (IDa)/1(1 freq.) -> iDa1/1
  phasor-magnitude (IDa)/2(2 freq.) -> iDa2/1
  phasor-magnitude (IDa)/3(5 freq.) -> iDa5/1
  Differential and restraining currents/4(iDb1) -> phasor-magnitude (iDb)/1(In1)
  Differential and restraining currents/5(iDb2) -> phasor-magnitude (iDb)/2(In2)
  Differential and restraining currents/6(iDb5) -> phasor-magnitude (iDb)/3(In3)
  phasor-magnitude (iDb)/1(1 freq.) -> iDb1/1
  phasor-magnitude (iDb)/2(2 freq.) -> iDb2/1
  phasor-magnitude (iDb)/3(5 freq.) -> iDb5/1
  Differential and restraining currents/7(iDc1) -> phasor-magnitude (iDc)/1(In1)
  Differential and restraining currents/8(iDc2) -> phasor-magnitude (iDc)/2(In2)
  Differential and restraining currents/9(iDc5) -> phasor-magnitude (iDc)/3(In3)
  phasor-magnitude (iDc)/1(1 freq.) -> iDc1/1
  phasor-magnitude (iDc)/2(2 freq.) -> iDc2/1
  phasor-magnitude (iDc)/3(5 freq.) -> iDc5/1
  Differential and restraining currents/10(iRa1) -> Phasor-magnitude (IR)/1(IRa1)
  Differential and restraining currents/11(iRb1) -> Phasor-magnitude (IR)/2(IRb1)
  Differential and restraining currents/12(iRc1) -> Phasor-magnitude (IR)/3(IRC1)
  Phasor-magnitude (IR)/1(1 freq.) -> iRa1/1
  Phasor-magnitude (IR)/2(1 freq.1) -> iRb1/1
  Phasor-magnitude (IR)/3(1 freq.2) -> iRc1/1

== system Copy_of_FaultFeeder/SM_WT1/Wind Type IV Detailed v2.1 - 1/AC fault ride though characteristic ==
  note: If more than X seconds under
      | FRT then disconnection message
  Va pu mag : Inport
  I 3ph pu : Inport  Port=2
  Compare To Constant : simulink/Logic and Bit Operations/Compare To Constant  relop=>=  const=Fault_Base_Duration_time_FRT  OutDataTypeStr=boolean
  Compare To Constant1 : simulink/Logic and Bit Operations/Compare To Constant  relop=<  const=0.2  OutDataTypeStr=boolean
  Compare To Constant2 : simulink/Logic and Bit Operations/Compare To Constant  relop=<  const=0.2  OutDataTypeStr=boolean
  Compare To Constant3 : simulink/Logic and Bit Operations/Compare To Constant  relop=<  const=0.5  OutDataTypeStr=boolean
  Constant : Constant  Value=0  SampleTime=Ts
  Constant1 : Constant  SampleTime=Ts
  Constant2 : Constant  Value=0  SampleTime=Ts
  Constant3 : Constant  Value=0
  Constant4 : Constant  Value=0
  Constant5 : Constant  Value=0
  Constant6 : Constant  Value=0.9  SampleTime=Ts
  Data Type Conversion : DataTypeConversion  OutDataTypeStr=double
  Digital Clock{1..4} (4 alike) : DigitalClock  SampleTime=Ts
  Discrete-Time Integrator : DiscreteIntegrator  ExternalReset=rising  SampleTime=Ts  ICPrevOutput=DiscIntNeverNeededParam  ICPrevScaledInput=DiscIntNeverNeededParam
  Memory : Memory
  MinMax : MinMax  Function=max
  MinMax Running Resettable : simulink/Math Operations/MinMax Running Resettable  Function=max  vinit=0.0
  MinMax Running Resettable1 : simulink/Math Operations/MinMax Running Resettable  Function=min  vinit=1
  MinMax Running Resettable2 : simulink/Math Operations/MinMax Running Resettable  Function=max  vinit=0.0
  MinMax1 : MinMax  Function=max
  MinMax2 : MinMax
  NOT : Logic  Operator=NOT  AllPortsSameDT=off  OutDataTypeStr=boolean
  OR : Logic  Operator=OR  AllPortsSameDT=off  OutDataTypeStr=boolean
  Relational Operator : RelationalOperator  Operator=<  OutDataTypeStr=boolean  RndMeth=Simplest
  "Sinusoidal Measurement (PLL, Three-Phase)1" : eeSinusoidalMeasurement/Sinusoidal Measurement (PLL, Three-Phase)  Kp_LF=200  Ki_LF=2000  F0=freq  Theta0=0  Ts=Ts
      settings: SourceProductBaseCode=PS
  Switch1 : Switch  Criteria=u2 > Threshold
  Switch2 : Switch  Criteria=u2 > Threshold
  Switch3 : Switch  Criteria=u2 > Threshold
  Terminator : Terminator
  Terminator1 : Terminator
  Triggered Subsystem : Subsystem  TreatAsAtomicUnit=on
  Disconnection_trigger : Outport  VectorParamsAs1DForOutWhenUnconnected=on
  Time_under_FRT : Outport  Port=2  VectorParamsAs1DForOutWhenUnconnected=on
  Min_voltage : Outport  Port=3  VectorParamsAs1DForOutWhenUnconnected=on
  Max_current : Outport  Port=4  VectorParamsAs1DForOutWhenUnconnected=on
  Time_trigger_FRT : Outport  Port=5  VectorParamsAs1DForOutWhenUnconnected=on
  wires:
  Data Type Conversion/1 -> Disconnection_trigger/1
  Constant5/1 -> MinMax Running Resettable2/2
  Constant4/1 -> MinMax Running Resettable1/2
  Constant3/1 -> MinMax Running Resettable/2
  MinMax2/1 -> MinMax Running Resettable1/1
  Switch3/1 -> MinMax2/1
  Switch1/1 -> MinMax1/1
  Compare To Constant2/1 -> Switch1/2
  Constant2/1 -> Switch1/1
  Digital Clock4/1 -> Compare To Constant2/1
  Triggered Subsystem/1(Time_trigger_FRT) -> Time_trigger_FRT/1
  Digital Clock3/1 -> Triggered Subsystem/1(In1)
  Digital Clock2/1 -> Compare To Constant1/1
  Constant1/1 -> Switch3/1
  Compare To Constant1/1 -> Switch3/2
  MinMax Running Resettable1/1 -> Min_voltage/1
  "Sinusoidal Measurement (PLL, Three-Phase)1"/1 -> Terminator1/1
  "Sinusoidal Measurement (PLL, Three-Phase)1"/2 -> Terminator/1
  "Sinusoidal Measurement (PLL, Three-Phase)1"/3 -> Switch1/3  "Vabc_pu_mag"
  I 3ph pu/1 -> "Sinusoidal Measurement (PLL, Three-Phase)1"/1
  MinMax Running Resettable2/1 -> Max_current/1
  MinMax1/1 -> MinMax Running Resettable2/1
  Va pu mag/1 -> Switch3/3, Relational Operator/1
  MinMax Running Resettable/1 -> Time_under_FRT/1
  MinMax/1 -> MinMax Running Resettable/1
  Memory/1 -> OR/1
  Compare To Constant/1 -> OR/2
  OR/1 -> Memory/1, Data Type Conversion/1, Triggered Subsystem/Trigger  "Disconnection_Trigger"
  NOT/1 -> Discrete-Time Integrator/2
  Switch2/1 -> Discrete-Time Integrator/1, NOT/1  "Va comparison to Vgrid"
  Constant/1 -> Switch2/1
  Compare To Constant3/1 -> Switch2/2
  Relational Operator/1 -> Switch2/3
  Digital Clock1/1 -> Compare To Constant3/1
  Discrete-Time Integrator/1 -> MinMax/1, Compare To Constant/1  "Integrator output"
  Constant6/1 -> Relational Operator/2
